simulink model "circuit"  (R2012b)
settings: Solver=ode45  StartTime=0.0  StopTime=10.0  RelTol=1e-3
settings Model: Creator=roberto  LastModifiedBy=roberto

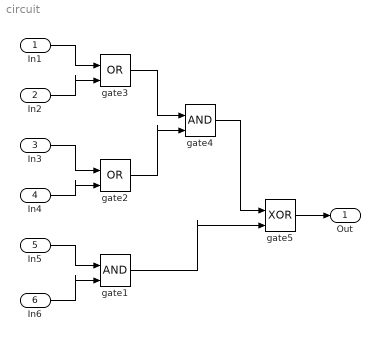
== system circuit ==
  In1 : Inport  OutDataTypeStr=boolean
  In2 : Inport  Port=2  OutDataTypeStr=boolean
  In3 : Inport  Port=3  OutDataTypeStr=boolean
  In4 : Inport  Port=4  OutDataTypeStr=boolean
  In5 : Inport  Port=5  OutDataTypeStr=boolean
  In6 : Inport  Port=6  OutDataTypeStr=boolean
  gate1 : Logic  IconShape=distinctive  AllPortsSameDT=off  OutDataTypeStr=boolean
  gate2 : Logic  Operator=OR  IconShape=distinctive  AllPortsSameDT=off  OutDataTypeStr=boolean
  gate3 : Logic  Operator=OR  IconShape=distinctive  AllPortsSameDT=off  OutDataTypeStr=boolean
  gate4 : Logic  IconShape=distinctive  AllPortsSameDT=off  OutDataTypeStr=boolean
  gate5 : Logic  Operator=XOR  IconShape=distinctive  AllPortsSameDT=off  OutDataTypeStr=boolean
  Out : Outport
  wires:
  In5/1 -> gate1/1
  In6/1 -> gate1/2
  In1/1 -> gate3/1
  In2/1 -> gate3/2
  In3/1 -> gate2/1
  In4/1 -> gate2/2
  gate3/1 -> gate4/1
  gate2/1 -> gate4/2
  gate4/1 -> gate5/1
  gate1/1 -> gate5/2
  gate5/1 -> Out/1
